simulink model "mrefrobotarm_previous_y_previous_u_previous_ref_cex_3b_breach"  (R2018b)
settings: Solver=FixedStepAuto  StartTime=0.0  StopTime=tspan(end)  RelTol=1e-3  AbsTol=1e-6
undefined symbols (not defined in the file): cc, options
libraries: neural x462, simulink x2
(part 6 of 18)

== system mrefrobotarm_previous_y_previous_u_previous_ref_cex_3b_breach/1000_epoch/Layer 3/Delays 1 ==
  "p{3}" : Inport  PortDimensions=30
      mask Display: e = 0.06;c1 = [120 230 180]/255;c2 = ([120 230 180]+0)/(256+128);c3 = ([120 230 180]+128)/(256+128);patch([0 1 1 0],[0 0 1 1],c1);patch([0 1 1 1-e 1-e 0+e],[0 0 1 1-e 0+e 0+e],c2);patch([0 0 1 1-e 0+e 0+e],[0 1 1 1-e 1-e 0+e],c3);plot([0 1 1 0 0],[0 0 1 1 0]);
  mux : Mux  Inputs=1
      mask Display: e = 0.06;c1 = [120 150 230]/255;c2 = ([120 150 230]+0)/383;c3 = ([120 150 230]+128)/383;patch([0 1 1 0],[0 0 1 1],c1);patch([0 1 1 1-e 1-e 0+e],[0 0 1 1-e 0+e 0+e],c2);patch([0 0 1 1-e 0+e 0+e],[0 1 1 1-e 1-e 0+e],c3);plot([0 1 1 0 0],[0 0 1 1 0]);disp('Mux')
  "pd{3,2}" : Outport
      mask Display: e = 0.06;c1 = [120 230 180]/255;c2 = ([120 230 180]+0)/(256+128);c3 = ([120 230 180]+128)/(256+128);patch([0 1 1 0],[0 0 1 1],c1);patch([0 1 1 1-e 1-e 0+e],[0 0 1 1-e 0+e 0+e],c2);patch([0 0 1 1-e 0+e 0+e],[0 1 1 1-e 1-e 0+e],c3);plot([0 1 1 0 0],[0 0 1 1 0]);
  wires:
  "p{3}"/1 -> mux/1
  mux/1 -> "pd{3,2}"/1

== system mrefrobotarm_previous_y_previous_u_previous_ref_cex_3b_breach/1000_epoch/Layer 3/LW{3,2} ==
  "ad{3,2}" : Inport  PortDimensions=30
      mask Display: e = 0.06;c1 = [120 230 180]/255;c2 = ([120 230 180]+0)/(256+128);c3 = ([120 230 180]+128)/(256+128);patch([0 1 1 0],[0 0 1 1],c1);patch([0 1 1 1-e 1-e 0+e],[0 0 1 1-e 0+e 0+e],c2);patch([0 0 1 1-e 0+e 0+e],[0 1 1 1-e 1-e 0+e],c3);plot([0 1 1 0 0],[0 0 1 1 0]);
  "IW{3,2}(1,:)'" : Constant  Value=[0.11985875790449669608950244992229272611439228057861328125;-0.33809477354095218704088665617746300995349884033203125;-0.94183273738662653951081438208348117768764495849609375;0.89870798994347789179215624244534410536289215087890625;0.2012965062689739681456302378137479536235332489013671875;-0.399237013762767489755134420192916877567768096923828125;-0.25175844333899777272023356999852694571018218994140625;-0.84683335263539960546808060826151631772518157958984375;0.397071945285334571007496151651139371097087860107421875;-0.04577368568539068316436413397241267375648021697998046875;-0.2301951027200161703500924659238080494105815887451171875;-0.03359406609631777895774717990207136608660221099853515625;0.060299848424656334044957617379623115994036197662353515625;0.65479640585044329714747846082900650799274444580078125;-0.0518272457760874660781524880803772248327732086181640625;-0.370720768865431982153069156993296928703784942626953125;0.306525432139559683708540660518337972462177276611328125;0.58896241532574344912376318461610935628414154052734375;0.78121017312365415019570491494960151612758636474609375;-0.380696291181496671018891220228397287428379058837890625;0.41463633045046421887747101209242828190326690673828125;0.442725554303413149082047084448277018964290618896484375;0.1274037416834881975002957688047899864614009857177734375;-0.52073392659884498723243950735195539891719818115234375;-0.10778374768362937452526040260636364109814167022705078125;0.1326681217256966138773321972621488384902477264404296875;0.0234221269442529377025064007966648205183446407318115234375;-0.63601271474577181219700605652178637683391571044921875;-0.31815600682753963912574590722215361893177032470703125;0.196772051900301503390977586605004034936428070068359375]
      mask Display: e = 0.06;c1 = [120 150 230]/255;c2 = ([120 150 230]+0)/383;c3 = ([120 150 230]+128)/383;patch([0 1 1 0],[0 0 1 1],c1);patch([0 1 1 1-e 1-e 0+e],[0 0 1 1-e 0+e 0+e],c2);patch([0 0 1 1-e 0+e 0+e],[0 1 1 1-e 1-e 0+e],c3);plot([0 1 1 0 0],[0 0 1 1 0]);disp('weights');
  Mux : Mux  Inputs=1
      mask Display: e = 0.06;c1 = [120 150 230]/255;c2 = ([120 150 230]+0)/383;c3 = ([120 150 230]+128)/383;patch([0 1 1 0],[0 0 1 1],c1);patch([0 1 1 1-e 1-e 0+e],[0 0 1 1-e 0+e 0+e],c2);patch([0 0 1 1-e 0+e 0+e],[0 1 1 1-e 1-e 0+e],c3);plot([0 1 1 0 0],[0 0 1 1 0]);disp('Mux');
  dotprod1 : neural/Weight Functions/dotprod
  "lz{3,2}" : Outport
      mask Display: e = 0.06;c1 = [120 230 180]/255;c2 = ([120 230 180]+0)/(256+128);c3 = ([120 230 180]+128)/(256+128);patch([0 1 1 0],[0 0 1 1],c1);patch([0 1 1 1-e 1-e 0+e],[0 0 1 1-e 0+e 0+e],c2);patch([0 0 1 1-e 0+e 0+e],[0 1 1 1-e 1-e 0+e],c3);plot([0 1 1 0 0],[0 0 1 1 0]);
  wires:
  "IW{3,2}(1,:)'"/1 -> dotprod1/1
  "ad{3,2}"/1 -> dotprod1/2
  dotprod1/1 -> Mux/1
  Mux/1 -> "lz{3,2}"/1

== system mrefrobotarm_previous_y_previous_u_previous_ref_cex_3b_breach/15000 epoch/Layer 1/Delays 1 ==
  "p{1}" : Inport  PortDimensions=10
      mask Display: e = 0.06;c1 = [120 230 180]/255;c2 = ([120 230 180]+0)/(256+128);c3 = ([120 230 180]+128)/(256+128);patch([0 1 1 0],[0 0 1 1],c1);patch([0 1 1 1-e 1-e 0+e],[0 0 1 1-e 0+e 0+e],c2);patch([0 0 1 1-e 0+e 0+e],[0 1 1 1-e 1-e 0+e],c3);plot([0 1 1 0 0],[0 0 1 1 0]);
  mux : Mux  Inputs=1
      mask Display: e = 0.06;c1 = [120 150 230]/255;c2 = ([120 150 230]+0)/383;c3 = ([120 150 230]+128)/383;patch([0 1 1 0],[0 0 1 1],c1);patch([0 1 1 1-e 1-e 0+e],[0 0 1 1-e 0+e 0+e],c2);patch([0 0 1 1-e 0+e 0+e],[0 1 1 1-e 1-e 0+e],c3);plot([0 1 1 0 0],[0 0 1 1 0]);disp('Mux')
  "pd{1,1}" : Outport
      mask Display: e = 0.06;c1 = [120 230 180]/255;c2 = ([120 230 180]+0)/(256+128);c3 = ([120 230 180]+128)/(256+128);patch([0 1 1 0],[0 0 1 1],c1);patch([0 1 1 1-e 1-e 0+e],[0 0 1 1-e 0+e 0+e],c2);patch([0 0 1 1-e 0+e 0+e],[0 1 1 1-e 1-e 0+e],c3);plot([0 1 1 0 0],[0 0 1 1 0]);
  wires:
  "p{1}"/1 -> mux/1
  mux/1 -> "pd{1,1}"/1

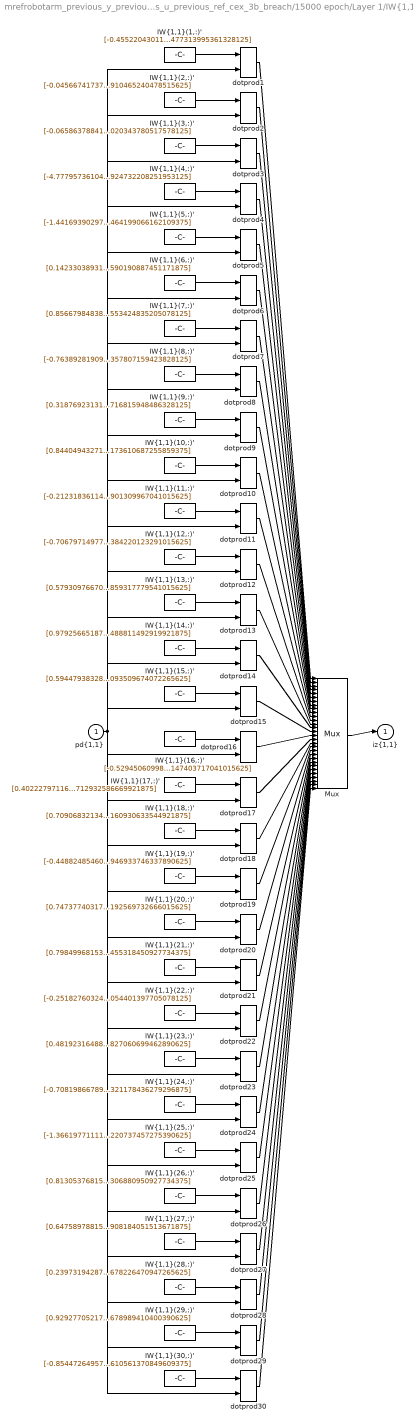
== system mrefrobotarm_previous_y_previous_u_previous_ref_cex_3b_breach/15000 epoch/Layer 1/IW{1,1} ==
  "pd{1,1}" : Inport  PortDimensions=10
      mask Display: e = 0.06;c1 = [120 230 180]/255;c2 = ([120 230 180]+0)/(256+128);c3 = ([120 230 180]+128)/(256+128);patch([0 1 1 0],[0 0 1 1],c1);patch([0 1 1 1-e 1-e 0+e],[0 0 1 1-e 0+e 0+e],c2);patch([0 0 1 1-e 0+e 0+e],[0 1 1 1-e 1-e 0+e],c3);plot([0 1 1 0 0],[0 0 1 1 0]);
  "IW{1,1}(1,:)'" : Constant  Value=[-0.455220430114593843651249471804476343095302581787109375;-2.10620377863470054080607951618731021881103515625;-0.479868449225107129851863874137052334845066070556640625;1.0055610598125543919678648308035917580127716064453125;-0.75734700576275770789180796782602556049823760986328125;0.3469225011322449869766160190920345485210418701171875;0.81470036038483695239875714833033271133899688720703125;0.4041870233089308594998101398232392966747283935546875;-0.6579959491618894151798713210155256092548370361328125;1.32415030494195651300515237380750477313995361328125]
      mask Display: e = 0.06;c1 = [120 150 230]/255;c2 = ([120 150 230]+0)/383;c3 = ([120 150 230]+128)/383;patch([0 1 1 0],[0 0 1 1],c1);patch([0 1 1 1-e 1-e 0+e],[0 0 1 1-e 0+e 0+e],c2);patch([0 0 1 1-e 0+e 0+e],[0 1 1 1-e 1-e 0+e],c3);plot([0 1 1 0 0],[0 0 1 1 0]);disp('Weights');
  "IW{1,1}(10,:)'" : Constant  Value=[0.8440494327199876689604707280523143708705902099609375;-0.75013572392803584687470674907672218978404998779296875;-0.265104932769315848606339613979798741638660430908203125;-0.7689187283703369235610125542734749615192413330078125;-0.1810488594997564371080756018272950313985347747802734375;0.2144663990194851932447051012786687351763248443603515625;-0.493659953379130322925760765429004095494747161865234375;0.433222827835198109891479134603287093341350555419921875;-1.15179403162659355075447820127010345458984375;0.06735814200090073367022114325664006173610687255859375]
      mask Display: e = 0.06;c1 = [120 150 230]/255;c2 = ([120 150 230]+0)/383;c3 = ([120 150 230]+128)/383;patch([0 1 1 0],[0 0 1 1],c1);patch([0 1 1 1-e 1-e 0+e],[0 0 1 1-e 0+e 0+e],c2);patch([0 0 1 1-e 0+e 0+e],[0 1 1 1-e 1-e 0+e],c3);plot([0 1 1 0 0],[0 0 1 1 0]);disp('Weights');
  "IW{1,1}(11,:)'" : Constant  Value=[-0.2123183611454251551453609181407955475151538848876953125;-0.340333467968539971071351146747474558651447296142578125;-0.443583736600105138503380430847755633294582366943359375;0.72334868961979548185325938902678899466991424560546875;-0.5038262209145483172534341065329499542713165283203125;0.04804101737326076093648197229413199238479137420654296875;-0.8549393641753602057775651701376773416996002197265625;0.57852733765980435265419146162457764148712158203125;-1.3565740262311105635006924785557202994823455810546875;-0.94499091422554271080258558868081308901309967041015625]
      mask Display: e = 0.06;c1 = [120 150 230]/255;c2 = ([120 150 230]+0)/383;c3 = ([120 150 230]+128)/383;patch([0 1 1 0],[0 0 1 1],c1);patch([0 1 1 1-e 1-e 0+e],[0 0 1 1-e 0+e 0+e],c2);patch([0 0 1 1-e 0+e 0+e],[0 1 1 1-e 1-e 0+e],c3);plot([0 1 1 0 0],[0 0 1 1 0]);disp('Weights');
  "IW{1,1}(12,:)'" : Constant  Value=[-0.70679714977365104555673269715043716132640838623046875;-0.05059830790756557339360455216592526994645595550537109375;0.2223031420607514407894456098802038468420505523681640625;0.63736910832481619149092466614092700183391571044921875;0.5939369807378287458021759448456577956676483154296875;0.7864089508551277418746394687332212924957275390625;0.42232861107089691987681590035208500921726226806640625;-0.347563836113860158416599688280257396399974822998046875;-0.6305941077264802796520370975486002862453460693359375;0.7645404458305391504069348229677416384220123291015625]
      mask Display: e = 0.06;c1 = [120 150 230]/255;c2 = ([120 150 230]+0)/383;c3 = ([120 150 230]+128)/383;patch([0 1 1 0],[0 0 1 1],c1);patch([0 1 1 1-e 1-e 0+e],[0 0 1 1-e 0+e 0+e],c2);patch([0 0 1 1-e 0+e 0+e],[0 1 1 1-e 1-e 0+e],c3);plot([0 1 1 0 0],[0 0 1 1 0]);disp('Weights');
  "IW{1,1}(13,:)'" : Constant  Value=[0.57930976670779943393796429518260993063449859619140625;-0.471575776761886167331994101914460770785808563232421875;-0.35435379859358173693095750422799028456211090087890625;-0.0032119351242606460072881446876635891385376453399658203125;1.1897578306314977591995329930796287953853607177734375;-0.277914872173078142392199652022100053727626800537109375;-0.52909292294290255487254626132198609411716461181640625;-0.85445810732122928765619462865288369357585906982421875;1.379693295673289465952393584302626550197601318359375;0.41914642500654564205575525193125940859317779541015625]
      mask Display: e = 0.06;c1 = [120 150 230]/255;c2 = ([120 150 230]+0)/383;c3 = ([120 150 230]+128)/383;patch([0 1 1 0],[0 0 1 1],c1);patch([0 1 1 1-e 1-e 0+e],[0 0 1 1-e 0+e 0+e],c2);patch([0 0 1 1-e 0+e 0+e],[0 1 1 1-e 1-e 0+e],c3);plot([0 1 1 0 0],[0 0 1 1 0]);disp('Weights');
  "IW{1,1}(14,:)'" : Constant  Value=[0.9792566518726701918495791687746532261371612548828125;0.1344833068538720255435947592559386976063251495361328125;0.4540267418923715769807358810794539749622344970703125;-0.2053468146119238613156454675845452584326267242431640625;-0.297814008008706776475804645087919197976589202880859375;0.26071633537487393095233301210100762546062469482421875;0.400753177313971920003865534454234875738620758056640625;1.126847525056398513498834290658123791217803955078125;0.314359572845778700855845499972929246723651885986328125;0.599630619426398947524603499914519488811492919921875]
      mask Display: e = 0.06;c1 = [120 150 230]/255;c2 = ([120 150 230]+0)/383;c3 = ([120 150 230]+128)/383;patch([0 1 1 0],[0 0 1 1],c1);patch([0 1 1 1-e 1-e 0+e],[0 0 1 1-e 0+e 0+e],c2);patch([0 0 1 1-e 0+e 0+e],[0 1 1 1-e 1-e 0+e],c3);plot([0 1 1 0 0],[0 0 1 1 0]);disp('Weights');
  "IW{1,1}(15,:)'" : Constant  Value=[0.59447938328892069304032474974519573152065277099609375;1.161708710561853319376268700580112636089324951171875;-0.2257581841016106649622230406748712994158267974853515625;0.3478685694476844059153108901227824389934539794921875;0.98811918866942105577066968180588446557521820068359375;-0.78474302280412810972620718530379235744476318359375;-0.66253315104040277905284028747701086103916168212890625;0.4597476567831260130247983397566713392734527587890625;-0.4669834526330112201009114869520999491214752197265625;0.451129005100296132102499768734560348093509674072265625]
      mask Display: e = 0.06;c1 = [120 150 230]/255;c2 = ([120 150 230]+0)/383;c3 = ([120 150 230]+128)/383;patch([0 1 1 0],[0 0 1 1],c1);patch([0 1 1 1-e 1-e 0+e],[0 0 1 1-e 0+e 0+e],c2);patch([0 0 1 1-e 0+e 0+e],[0 1 1 1-e 1-e 0+e],c3);plot([0 1 1 0 0],[0 0 1 1 0]);disp('Weights');
  "IW{1,1}(16,:)'" : Constant  Value=[-0.52945060998214621417190528518403880298137664794921875;0.38286682603327604201837175423861481249332427978515625;-0.69768586754663142190935332109802402555942535400390625;-0.2251407366045608260396448940809932537376880645751953125;-0.67850401060618159565507312436238862574100494384765625;-0.82530949350363591587864675602759234607219696044921875;-0.313183019700349396519101219382719136774539947509765625;-0.85202914816623998017774965774151496589183807373046875;0.244475951486091191977578773730783723294734954833984375;-0.541679750908939272591169356019236147403717041015625]
      mask Display: e = 0.06;c1 = [120 150 230]/255;c2 = ([120 150 230]+0)/383;c3 = ([120 150 230]+128)/383;patch([0 1 1 0],[0 0 1 1],c1);patch([0 1 1 1-e 1-e 0+e],[0 0 1 1-e 0+e 0+e],c2);patch([0 0 1 1-e 0+e 0+e],[0 1 1 1-e 1-e 0+e],c3);plot([0 1 1 0 0],[0 0 1 1 0]);disp('Weights');
  "IW{1,1}(17,:)'" : Constant  Value=[0.40222797116094088920590365887619554996490478515625;0.7220732043634203733972753980197012424468994140625;-0.9741249830487370697795768137439154088497161865234375;0.394031575178730941733107329127960838377475738525390625;-0.3924287947518088071063857569242827594280242919921875;-0.47475713928896812188185094782966189086437225341796875;-0.443583220694766022784705228332313708961009979248046875;0.2280641254112396876241319887412828393280506134033203125;-0.1353233712787080822437246752087958157062530517578125;1.121005217616392268809022425557486712932586669921875]
      mask Display: e = 0.06;c1 = [120 150 230]/255;c2 = ([120 150 230]+0)/383;c3 = ([120 150 230]+128)/383;patch([0 1 1 0],[0 0 1 1],c1);patch([0 1 1 1-e 1-e 0+e],[0 0 1 1-e 0+e 0+e],c2);patch([0 0 1 1-e 0+e 0+e],[0 1 1 1-e 1-e 0+e],c3);plot([0 1 1 0 0],[0 0 1 1 0]);disp('Weights');
  "IW{1,1}(18,:)'" : Constant  Value=[0.7090683213481785429621595540083944797515869140625;0.45314535347316409197304665212868712842464447021484375;0.826518895367450046052226753090508282184600830078125;0.376618709326007550242110255567240528762340545654296875;-0.5007379362778616727069902481161989271640777587890625;-0.33012382423814246035220776320784352719783782958984375;-0.71692583599511727765474233819986693561077117919921875;-0.896291255931064512196826399303972721099853515625;2.0880157859334804726358925108797848224639892578125;1.1073921013793324163998477160930633544921875]
      mask Display: e = 0.06;c1 = [120 150 230]/255;c2 = ([120 150 230]+0)/383;c3 = ([120 150 230]+128)/383;patch([0 1 1 0],[0 0 1 1],c1);patch([0 1 1 1-e 1-e 0+e],[0 0 1 1-e 0+e 0+e],c2);patch([0 0 1 1-e 0+e 0+e],[0 1 1 1-e 1-e 0+e],c3);plot([0 1 1 0 0],[0 0 1 1 0]);disp('Weights');
  "IW{1,1}(19,:)'" : Constant  Value=[-0.44882485460073129335256680860766209661960601806640625;-0.1712058963567985869769216833446989767253398895263671875;-0.71925696260688376515446407211129553616046905517578125;0.438778794759695445204528141402988694608211517333984375;0.4475733002654800340991414486779831349849700927734375;0.21975162674826143049955362585023976862430572509765625;-0.9626586586878100870734442651155404746532440185546875;0.158735943708872506707763250233256258070468902587890625;1.0468634120891195937730344667215831577777862548828125;0.33202427037668125198166535483323968946933746337890625]
      mask Display: e = 0.06;c1 = [120 150 230]/255;c2 = ([120 150 230]+0)/383;c3 = ([120 150 230]+128)/383;patch([0 1 1 0],[0 0 1 1],c1);patch([0 1 1 1-e 1-e 0+e],[0 0 1 1-e 0+e 0+e],c2);patch([0 0 1 1-e 0+e 0+e],[0 1 1 1-e 1-e 0+e],c3);plot([0 1 1 0 0],[0 0 1 1 0]);disp('Weights');
  "IW{1,1}(2,:)'" : Constant  Value=[-0.045667417373742531794267307532209088094532489776611328125;0.80860551366365196468422027464839629828929901123046875;0.62592060196800602955846670738537795841693878173828125;-1.3579271334625406808527259272523224353790283203125;0.449980626343166267844253525254316627979278564453125;-0.54845161193768598995035290499799884855747222900390625;-0.05519885597823871725697841839064494706690311431884765625;-0.7070314258564660558903369746985845267772674560546875;-1.681879350398180594794439457473345100879669189453125;-0.85912502336537655001080793226719833910465240478515625]
      mask Display: e = 0.06;c1 = [120 150 230]/255;c2 = ([120 150 230]+0)/383;c3 = ([120 150 230]+128)/383;patch([0 1 1 0],[0 0 1 1],c1);patch([0 1 1 1-e 1-e 0+e],[0 0 1 1-e 0+e 0+e],c2);patch([0 0 1 1-e 0+e 0+e],[0 1 1 1-e 1-e 0+e],c3);plot([0 1 1 0 0],[0 0 1 1 0]);disp('Weights');
  "IW{1,1}(20,:)'" : Constant  Value=[0.7473774031764783831732756880228407680988311767578125;0.92032778951639337972068233284517191350460052490234375;-0.2990936874426435299056947769713588058948516845703125;1.1636059685250803585887524604913778603076934814453125;-0.399320700549953666591562750909361056983470916748046875;1.1084952037977731098550293609150685369968414306640625;0.84550302083813344555807134383940137922763824462890625;1.39836064663870818236546256230212748050689697265625;0.042768035257423904493823130223972839303314685821533203125;0.10289334014099939251796200778699130751192569732666015625]
      mask Display: e = 0.06;c1 = [120 150 230]/255;c2 = ([120 150 230]+0)/383;c3 = ([120 150 230]+128)/383;patch([0 1 1 0],[0 0 1 1],c1);patch([0 1 1 1-e 1-e 0+e],[0 0 1 1-e 0+e 0+e],c2);patch([0 0 1 1-e 0+e 0+e],[0 1 1 1-e 1-e 0+e],c3);plot([0 1 1 0 0],[0 0 1 1 0]);disp('Weights');
  "IW{1,1}(21,:)'" : Constant  Value=[0.79849968153554906624691511751734651625156402587890625;0.1577100102995146191364739252094295807182788848876953125;0.84639538122070778758399001162615604698657989501953125;0.616664395780805563163085025735199451446533203125;-0.08463400666176286446518162165375542826950550079345703125;-0.50657767441101742011966280188062228262424468994140625;-0.1347424116844726516006858219043351709842681884765625;0.7853093162862558873626994682126678526401519775390625;-0.33679095868648467604344887149636633694171905517578125;-1.583249706214013396987638770951889455318450927734375]
      mask Display: e = 0.06;c1 = [120 150 230]/255;c2 = ([120 150 230]+0)/383;c3 = ([120 150 230]+128)/383;patch([0 1 1 0],[0 0 1 1],c1);patch([0 1 1 1-e 1-e 0+e],[0 0 1 1-e 0+e 0+e],c2);patch([0 0 1 1-e 0+e 0+e],[0 1 1 1-e 1-e 0+e],c3);plot([0 1 1 0 0],[0 0 1 1 0]);disp('Weights');
  "IW{1,1}(22,:)'" : Constant  Value=[-0.2518276032492032801002324049477465450763702392578125;1.3385158507353540624507104439544491469860076904296875;-0.1731200681158149567995252482432988472282886505126953125;1.1553195793800361546033172999159432947635650634765625;-0.60813808218563136787082612499943934381008148193359375;-0.04127254955108938805352636336465366184711456298828125;1.0137832552985788225896612857468426227569580078125;-0.09149833010123675780533858414855785667896270751953125;3.854198795296192248116540213231928646564483642578125;0.50895126082326946903577891134773381054401397705078125]
      mask Display: e = 0.06;c1 = [120 150 230]/255;c2 = ([120 150 230]+0)/383;c3 = ([120 150 230]+128)/383;patch([0 1 1 0],[0 0 1 1],c1);patch([0 1 1 1-e 1-e 0+e],[0 0 1 1-e 0+e 0+e],c2);patch([0 0 1 1-e 0+e 0+e],[0 1 1 1-e 1-e 0+e],c3);plot([0 1 1 0 0],[0 0 1 1 0]);disp('Weights');
  "IW{1,1}(23,:)'" : Constant  Value=[0.4819231648826278746611251335707493126392364501953125;-0.70814816982524864119596941236522980034351348876953125;0.63708271793506410229923631050041876733303070068359375;-0.35800344396326522211637666259775869548320770263671875;-1.070308938197412462756119566620327532291412353515625;0.0737815181466469904858485051590832881629467010498046875;-0.87674255370854170532624038969515822827816009521484375;-0.09173274010824740420932954521049396134912967681884765625;-0.7768544420155019114559991066926158964633941650390625;-0.86712247458394708932161165648722089827060699462890625]
      mask Display: e = 0.06;c1 = [120 150 230]/255;c2 = ([120 150 230]+0)/383;c3 = ([120 150 230]+128)/383;patch([0 1 1 0],[0 0 1 1],c1);patch([0 1 1 1-e 1-e 0+e],[0 0 1 1-e 0+e 0+e],c2);patch([0 0 1 1-e 0+e 0+e],[0 1 1 1-e 1-e 0+e],c3);plot([0 1 1 0 0],[0 0 1 1 0]);disp('Weights');
  "IW{1,1}(24,:)'" : Constant  Value=[-0.7081986678927816303286135735106654465198516845703125;-0.27598153385000834258988788860733620822429656982421875;-0.220317794960367463463768444853485561907291412353515625;-0.721538577371394485027167320367880165576934814453125;-0.7443257381787200532841097810887731611728668212890625;-0.8742112284211842609948917015572078526020050048828125;-0.85782768219084026828369360373471863567829132080078125;0.477106891531099919223635197340627200901508331298828125;1.013723137303741861359185350011102855205535888671875;-0.2305303420184771912015975203757989220321178436279296875]
      mask Display: e = 0.06;c1 = [120 150 230]/255;c2 = ([120 150 230]+0)/383;c3 = ([120 150 230]+128)/383;patch([0 1 1 0],[0 0 1 1],c1);patch([0 1 1 1-e 1-e 0+e],[0 0 1 1-e 0+e 0+e],c2);patch([0 0 1 1-e 0+e 0+e],[0 1 1 1-e 1-e 0+e],c3);plot([0 1 1 0 0],[0 0 1 1 0]);disp('Weights');
  "IW{1,1}(25,:)'" : Constant  Value=[-1.366197711118600555124658058048225939273834228515625;-0.2268951750901318231701253580467891879379749298095703125;-0.5575549725072945772552657217602245509624481201171875;-0.90648110489400668399184723966754972934722900390625;-0.46128629616771010812925624122726731002330780029296875;0.8011951497706604197190927152405492961406707763671875;-0.7907631640821737306623617769218981266021728515625;-0.309082292333055896893512226597522385418415069580078125;-0.004322454099595690081569987484044759185053408145904541015625;1.1149382021470390924378079944290220737457275390625]
      mask Display: e = 0.06;c1 = [120 150 230]/255;c2 = ([120 150 230]+0)/383;c3 = ([120 150 230]+128)/383;patch([0 1 1 0],[0 0 1 1],c1);patch([0 1 1 1-e 1-e 0+e],[0 0 1 1-e 0+e 0+e],c2);patch([0 0 1 1-e 0+e 0+e],[0 1 1 1-e 1-e 0+e],c3);plot([0 1 1 0 0],[0 0 1 1 0]);disp('Weights');
  "IW{1,1}(26,:)'" : Constant  Value=[0.813053768154178069238469106494449079036712646484375;0.4544848137708712432214497312088496983051300048828125;-0.6751735376907372909727200749330222606658935546875;0.362668257073277822133405834392760880291461944580078125;0.62482471301260422702483765533543191850185394287109375;-0.54025646345486288968373855823301710188388824462890625;-0.77869337605968180771043307686340995132923126220703125;0.55712251789180078365149029195890761911869049072265625;0.66692326371604881973809142436948604881763458251953125;-0.337863104277960013543946615754975937306880950927734375]
      mask Display: e = 0.06;c1 = [120 150 230]/255;c2 = ([120 150 230]+0)/383;c3 = ([120 150 230]+128)/383;patch([0 1 1 0],[0 0 1 1],c1);patch([0 1 1 1-e 1-e 0+e],[0 0 1 1-e 0+e 0+e],c2);patch([0 0 1 1-e 0+e 0+e],[0 1 1 1-e 1-e 0+e],c3);plot([0 1 1 0 0],[0 0 1 1 0]);disp('Weights');
  "IW{1,1}(27,:)'" : Constant  Value=[0.647589788158871471068778191693127155303955078125;-0.416930857377221519843857322484836913645267486572265625;0.773103229958802984356225351803004741668701171875;0.251904466038396446236902193049900233745574951171875;0.166622225078163987976864746087812818586826324462890625;-0.81226837724227951564870409129071049392223358154296875;-0.83715413550326556180181114541483111679553985595703125;0.9795946273618174604536079641547985374927520751953125;1.5469271226040011146807273689773865044116973876953125;2.190888857539163847576446642051450908184051513671875]
      mask Display: e = 0.06;c1 = [120 150 230]/255;c2 = ([120 150 230]+0)/383;c3 = ([120 150 230]+128)/383;patch([0 1 1 0],[0 0 1 1],c1);patch([0 1 1 1-e 1-e 0+e],[0 0 1 1-e 0+e 0+e],c2);patch([0 0 1 1-e 0+e 0+e],[0 1 1 1-e 1-e 0+e],c3);plot([0 1 1 0 0],[0 0 1 1 0]);disp('Weights');
  "IW{1,1}(28,:)'" : Constant  Value=[0.239731942879117643219188948933151550590991973876953125;0.82195825966009816720969638481619767844676971435546875;0.1087706803352469775436617283048690296709537506103515625;-0.57352744621838613880981938564218580722808837890625;-0.478309332616384919045771084711304865777492523193359375;-1.2731811989049004463225855943164788186550140380859375;-0.89490318176718719467288565283524803817272186279296875;0.11038680868376561650112677170909591950476169586181640625;-0.1986707997599289343693129694656818173825740814208984375;-0.43092275743799268727940443568513728678226470947265625]
      mask Display: e = 0.06;c1 = [120 150 230]/255;c2 = ([120 150 230]+0)/383;c3 = ([120 150 230]+128)/383;patch([0 1 1 0],[0 0 1 1],c1);patch([0 1 1 1-e 1-e 0+e],[0 0 1 1-e 0+e 0+e],c2);patch([0 0 1 1-e 0+e 0+e],[0 1 1 1-e 1-e 0+e],c3);plot([0 1 1 0 0],[0 0 1 1 0]);disp('Weights');
  "IW{1,1}(29,:)'" : Constant  Value=[0.92927705217238665280632403664640150964260101318359375;0.294715120235578054153080529431463219225406646728515625;-0.51596740047337663614968050751485861837863922119140625;-0.65702001933077713857755952631123363971710205078125;-0.7764423967805307302825212900643236935138702392578125;0.291167084777243234672283733743824996054172515869140625;0.541160979640257888689802712178789079189300537109375;0.281494097405528054256507175523438490927219390869140625;-2.9250126675494545480660235625691711902618408203125;-3.205456821109232468103300561779178678989410400390625]
      mask Display: e = 0.06;c1 = [120 150 230]/255;c2 = ([120 150 230]+0)/383;c3 = ([120 150 230]+128)/383;patch([0 1 1 0],[0 0 1 1],c1);patch([0 1 1 1-e 1-e 0+e],[0 0 1 1-e 0+e 0+e],c2);patch([0 0 1 1-e 0+e 0+e],[0 1 1 1-e 1-e 0+e],c3);plot([0 1 1 0 0],[0 0 1 1 0]);disp('Weights');
  "IW{1,1}(3,:)'" : Constant  Value=[-0.065863788414856350161841191948042251169681549072265625;0.037813680350472507474268724081412074156105518341064453125;0.8041676885649533534916599819553084671497344970703125;-0.818425645507755650243097989005036652088165283203125;-0.12413062803535819533795603319958900101482868194580078125;0.498314913424161343158402814879082143306732177734375;0.318343962723618478793952135674771852791309356689453125;-0.430522720929491564678670556531869806349277496337890625;1.81525495139902215413485464523546397686004638671875;2.9462204253596411263060872443020343780517578125]
      mask Display: e = 0.06;c1 = [120 150 230]/255;c2 = ([120 150 230]+0)/383;c3 = ([120 150 230]+128)/383;patch([0 1 1 0],[0 0 1 1],c1);patch([0 1 1 1-e 1-e 0+e],[0 0 1 1-e 0+e 0+e],c2);patch([0 0 1 1-e 0+e 0+e],[0 1 1 1-e 1-e 0+e],c3);plot([0 1 1 0 0],[0 0 1 1 0]);disp('Weights');
  "IW{1,1}(30,:)'" : Constant  Value=[-0.8544726495754051409647900072741322219371795654296875;-0.10053148502334945113556585738479043357074260711669921875;-0.88986220368823831794458101285272277891635894775390625;0.7666301471184997495811330736614763736724853515625;0.44707720129477623860481116935261525213718414306640625;0.204158672821065756419756098694051615893840789794921875;0.134429241483858763483993925547110848128795623779296875;-0.7099096358169572074103825798374600708484649658203125;0.49453127875069691210541122927679680287837982177734375;0.785488784995612032702183569199405610561370849609375]
      mask Display: e = 0.06;c1 = [120 150 230]/255;c2 = ([120 150 230]+0)/383;c3 = ([120 150 230]+128)/383;patch([0 1 1 0],[0 0 1 1],c1);patch([0 1 1 1-e 1-e 0+e],[0 0 1 1-e 0+e 0+e],c2);patch([0 0 1 1-e 0+e 0+e],[0 1 1 1-e 1-e 0+e],c3);plot([0 1 1 0 0],[0 0 1 1 0]);disp('Weights');
  "IW{1,1}(4,:)'" : Constant  Value=[-4.77795736104125001730835720081813633441925048828125;1.3763486014871972873407912629772908985614776611328125;0.021973572656453936591258724320141482166945934295654296875;0.1256707363845366298704675500630401074886322021484375;-0.97605097883110525369687593411072157323360443115234375;0.78621043598603390645251920432201586663722991943359375;-0.5349299608420354790183637305744923651218414306640625;-1.8588218662031101846565661617205478250980377197265625;-0.08670229135174410683983836634070030413568019866943359375;-0.642276748399158936564390387502498924732208251953125]
      mask Display: e = 0.06;c1 = [120 150 230]/255;c2 = ([120 150 230]+0)/383;c3 = ([120 150 230]+128)/383;patch([0 1 1 0],[0 0 1 1],c1);patch([0 1 1 1-e 1-e 0+e],[0 0 1 1-e 0+e 0+e],c2);patch([0 0 1 1-e 0+e 0+e],[0 1 1 1-e 1-e 0+e],c3);plot([0 1 1 0 0],[0 0 1 1 0]);disp('Weights');
  "IW{1,1}(5,:)'" : Constant  Value=[-1.4416939029743993661014656026964075863361358642578125;0.2783694158870504420377756105153821408748626708984375;-0.218466894654460508373716720598167739808559417724609375;-0.2387002443128883044654031664322246797382831573486328125;-0.381684455859159388335655194168793968856334686279296875;-0.7291095220461250026033894755528308451175689697265625;0.2414439969273430020013648800158989615738391876220703125;0.2270096458971715691621540145206381566822528839111328125;-3.460960245428166270897918366244994103908538818359375;0.472158477384735097981405260725296102464199066162109375]
      mask Display: e = 0.06;c1 = [120 150 230]/255;c2 = ([120 150 230]+0)/383;c3 = ([120 150 230]+128)/383;patch([0 1 1 0],[0 0 1 1],c1);patch([0 1 1 1-e 1-e 0+e],[0 0 1 1-e 0+e 0+e],c2);patch([0 0 1 1-e 0+e 0+e],[0 1 1 1-e 1-e 0+e],c3);plot([0 1 1 0 0],[0 0 1 1 0]);disp('Weights');
  "IW{1,1}(6,:)'" : Constant  Value=[0.142330389311283223019444221790763549506664276123046875;-1.188375461540883915034783058217726647853851318359375;0.85957045377895380244837042482686229050159454345703125;-0.259142390818316414868860420028795488178730010986328125;0.10847872467499790338774090514561976306140422821044921875;-0.499618438061193936849946339862071909010410308837890625;-1.0932708069397027994540394502109847962856292724609375;-0.0623255531112183458475328734493814408779144287109375;-0.1608528275658193396058237567558535374701023101806640625;0.646157980419090005597126946668140590190887451171875]
      mask Display: e = 0.06;c1 = [120 150 230]/255;c2 = ([120 150 230]+0)/383;c3 = ([120 150 230]+128)/383;patch([0 1 1 0],[0 0 1 1],c1);patch([0 1 1 1-e 1-e 0+e],[0 0 1 1-e 0+e 0+e],c2);patch([0 0 1 1-e 0+e 0+e],[0 1 1 1-e 1-e 0+e],c3);plot([0 1 1 0 0],[0 0 1 1 0]);disp('Weights');
  "IW{1,1}(7,:)'" : Constant  Value=[0.8566798483849951129087685330887325108051300048828125;0.81433221942370492829610384433181025087833404541015625;1.0856629828789101654962223619804717600345611572265625;-0.89740206988252513298220947035588324069976806640625;1.4380144031638817381235639913938939571380615234375;2.053074626354669529604279887280426919460296630859375;-0.399378528306981006590348215468111447989940643310546875;2.98958492216014892761677401722408831119537353515625;3.337110261684952394745096171391196548938751220703125;3.075365269144122226663284891401417553424835205078125]
      mask Display: e = 0.06;c1 = [120 150 230]/255;c2 = ([120 150 230]+0)/383;c3 = ([120 150 230]+128)/383;patch([0 1 1 0],[0 0 1 1],c1);patch([0 1 1 1-e 1-e 0+e],[0 0 1 1-e 0+e 0+e],c2);patch([0 0 1 1-e 0+e 0+e],[0 1 1 1-e 1-e 0+e],c3);plot([0 1 1 0 0],[0 0 1 1 0]);disp('Weights');
  "IW{1,1}(8,:)'" : Constant  Value=[-0.7638928190907610105142566681024618446826934814453125;-0.248208480751506865846778282502782531082630157470703125;0.3746661363550745083017545766779221594333648681640625;0.59669538903291263753914108747267164289951324462890625;0.0442144234440020322818298836864414624869823455810546875;-0.1755943159757873683890494476145249791443347930908203125;0.0675267461112324662853012569030397571623325347900390625;-0.7188665591787302133752746158279478549957275390625;-0.6144826943747145886476346277049742639064788818359375;-0.51773743660324200721589704698999412357807159423828125]
      mask Display: e = 0.06;c1 = [120 150 230]/255;c2 = ([120 150 230]+0)/383;c3 = ([120 150 230]+128)/383;patch([0 1 1 0],[0 0 1 1],c1);patch([0 1 1 1-e 1-e 0+e],[0 0 1 1-e 0+e 0+e],c2);patch([0 0 1 1-e 0+e 0+e],[0 1 1 1-e 1-e 0+e],c3);plot([0 1 1 0 0],[0 0 1 1 0]);disp('Weights');
  "IW{1,1}(9,:)'" : Constant  Value=[0.3187692313172199032322851053322665393352508544921875;1.546390735928829140988227663910947740077972412109375;0.9617053179127788009594723916961811482906341552734375;-1.5763561860234001077429866199963726103305816650390625;3.696204709767358043137619461049325764179229736328125;0.463426033588114461014839662311715073883533477783203125;-2.935127736394651520868137595243752002716064453125;-0.142428544528001743696421499407733790576457977294921875;3.547367165142917944109512973227538168430328369140625;0.9379049051031700390268497358192689716815948486328125]
      mask Display: e = 0.06;c1 = [120 150 230]/255;c2 = ([120 150 230]+0)/383;c3 = ([120 150 230]+128)/383;patch([0 1 1 0],[0 0 1 1],c1);patch([0 1 1 1-e 1-e 0+e],[0 0 1 1-e 0+e 0+e],c2);patch([0 0 1 1-e 0+e 0+e],[0 1 1 1-e 1-e 0+e],c3);plot([0 1 1 0 0],[0 0 1 1 0]);disp('Weights');
  Mux : Mux  Inputs=30
      mask Display: e = 0.06;c1 = [120 150 230]/255;c2 = ([120 150 230]+0)/383;c3 = ([120 150 230]+128)/383;patch([0 1 1 0],[0 0 1 1],c1);patch([0 1 1 1-e 1-e 0+e],[0 0 1 1-e 0+e 0+e],c2);patch([0 0 1 1-e 0+e 0+e],[0 1 1 1-e 1-e 0+e],c3);plot([0 1 1 0 0],[0 0 1 1 0]);disp('Mux');
  dotprod{1..30} (30 alike) : neural/Weight Functions/dotprod
  "iz{1,1}" : Outport
      mask Display: e = 0.06;c1 = [120 230 180]/255;c2 = ([120 230 180]+0)/(256+128);c3 = ([120 230 180]+128)/(256+128);patch([0 1 1 0],[0 0 1 1],c1);patch([0 1 1 1-e 1-e 0+e],[0 0 1 1-e 0+e 0+e],c2);patch([0 0 1 1-e 0+e 0+e],[0 1 1 1-e 1-e 0+e],c3);plot([0 1 1 0 0],[0 0 1 1 0]);
  wires:
  "IW{1,1}(1,:)'"/1 -> dotprod1/1
  "pd{1,1}"/1 -> dotprod1/2, dotprod2/2, dotprod3/2, dotprod4/2, dotprod5/2, dotprod6/2, dotprod7/2, dotprod8/2, dotprod9/2, dotprod10/2, dotprod11/2, dotprod12/2, dotprod13/2, dotprod14/2, dotprod15/2, dotprod16/2, dotprod17/2, dotprod18/2, dotprod19/2, dotprod20/2, dotprod21/2, dotprod22/2, dotprod23/2, dotprod24/2, dotprod25/2, dotprod26/2, dotprod27/2, dotprod28/2, dotprod29/2, dotprod30/2
  dotprod1/1 -> Mux/1
  "IW{1,1}(2,:)'"/1 -> dotprod2/1
  dotprod2/1 -> Mux/2
  "IW{1,1}(3,:)'"/1 -> dotprod3/1
  dotprod3/1 -> Mux/3
  "IW{1,1}(4,:)'"/1 -> dotprod4/1
  dotprod4/1 -> Mux/4
  "IW{1,1}(5,:)'"/1 -> dotprod5/1
  dotprod5/1 -> Mux/5
  "IW{1,1}(6,:)'"/1 -> dotprod6/1
  dotprod6/1 -> Mux/6
  "IW{1,1}(7,:)'"/1 -> dotprod7/1
  dotprod7/1 -> Mux/7
  "IW{1,1}(8,:)'"/1 -> dotprod8/1
  dotprod8/1 -> Mux/8
  "IW{1,1}(9,:)'"/1 -> dotprod9/1
  dotprod9/1 -> Mux/9
  "IW{1,1}(10,:)'"/1 -> dotprod10/1
  dotprod10/1 -> Mux/10
  "IW{1,1}(11,:)'"/1 -> dotprod11/1
  dotprod11/1 -> Mux/11
  "IW{1,1}(12,:)'"/1 -> dotprod12/1
  dotprod12/1 -> Mux/12
  "IW{1,1}(13,:)'"/1 -> dotprod13/1
  dotprod13/1 -> Mux/13
  "IW{1,1}(14,:)'"/1 -> dotprod14/1
  dotprod14/1 -> Mux/14
  "IW{1,1}(15,:)'"/1 -> dotprod15/1
  dotprod15/1 -> Mux/15
  "IW{1,1}(16,:)'"/1 -> dotprod16/1
  dotprod16/1 -> Mux/16
  "IW{1,1}(17,:)'"/1 -> dotprod17/1
  dotprod17/1 -> Mux/17
  "IW{1,1}(18,:)'"/1 -> dotprod18/1
  dotprod18/1 -> Mux/18
  "IW{1,1}(19,:)'"/1 -> dotprod19/1
  dotprod19/1 -> Mux/19
  "IW{1,1}(20,:)'"/1 -> dotprod20/1
  dotprod20/1 -> Mux/20
  "IW{1,1}(21,:)'"/1 -> dotprod21/1
  dotprod21/1 -> Mux/21
  "IW{1,1}(22,:)'"/1 -> dotprod22/1
  dotprod22/1 -> Mux/22
  "IW{1,1}(23,:)'"/1 -> dotprod23/1
  dotprod23/1 -> Mux/23
  "IW{1,1}(24,:)'"/1 -> dotprod24/1
  dotprod24/1 -> Mux/24
  "IW{1,1}(25,:)'"/1 -> dotprod25/1
  dotprod25/1 -> Mux/25
  "IW{1,1}(26,:)'"/1 -> dotprod26/1
  dotprod26/1 -> Mux/26
  "IW{1,1}(27,:)'"/1 -> dotprod27/1
  dotprod27/1 -> Mux/27
  "IW{1,1}(28,:)'"/1 -> dotprod28/1
  dotprod28/1 -> Mux/28
  "IW{1,1}(29,:)'"/1 -> dotprod29/1
  dotprod29/1 -> Mux/29
  "IW{1,1}(30,:)'"/1 -> dotprod30/1
  dotprod30/1 -> Mux/30
  Mux/1 -> "iz{1,1}"/1

== system mrefrobotarm_previous_y_previous_u_previous_ref_cex_3b_breach/15000 epoch/Layer 2/Delays 1 ==
  "p{2}" : Inport  PortDimensions=30
      mask Display: e = 0.06;c1 = [120 230 180]/255;c2 = ([120 230 180]+0)/(256+128);c3 = ([120 230 180]+128)/(256+128);patch([0 1 1 0],[0 0 1 1],c1);patch([0 1 1 1-e 1-e 0+e],[0 0 1 1-e 0+e 0+e],c2);patch([0 0 1 1-e 0+e 0+e],[0 1 1 1-e 1-e 0+e],c3);plot([0 1 1 0 0],[0 0 1 1 0]);
  mux : Mux  Inputs=1
      mask Display: e = 0.06;c1 = [120 150 230]/255;c2 = ([120 150 230]+0)/383;c3 = ([120 150 230]+128)/383;patch([0 1 1 0],[0 0 1 1],c1);patch([0 1 1 1-e 1-e 0+e],[0 0 1 1-e 0+e 0+e],c2);patch([0 0 1 1-e 0+e 0+e],[0 1 1 1-e 1-e 0+e],c3);plot([0 1 1 0 0],[0 0 1 1 0]);disp('Mux')
  "pd{2,1}" : Outport
      mask Display: e = 0.06;c1 = [120 230 180]/255;c2 = ([120 230 180]+0)/(256+128);c3 = ([120 230 180]+128)/(256+128);patch([0 1 1 0],[0 0 1 1],c1);patch([0 1 1 1-e 1-e 0+e],[0 0 1 1-e 0+e 0+e],c2);patch([0 0 1 1-e 0+e 0+e],[0 1 1 1-e 1-e 0+e],c3);plot([0 1 1 0 0],[0 0 1 1 0]);
  wires:
  "p{2}"/1 -> mux/1
  mux/1 -> "pd{2,1}"/1
